simulink model "MPC_Demo_wuguzhang"  (R2024a)
settings: Solver=ode1  StartTime=0.001  StopTime=16  FixedStep=0.001  RelTol=1e-3  EnableMultiTasking=on
model workspace (MAT data in the model file):
  cc = 10
libraries: simulink x3, SignalEditorBlockLib x3, Solver_SF x1, slpidlib x1
(part 5 of 5)

== matlab function MPC_Demo_wuguzhang/Controller/MATLAB Function ==
  data: Vx input; beta output; Vy input; omega_1 input; omega_2 input; omega_3 input; omega_4 input; lamda1 output; lamda2 output; lamda3 output; lamda4 output
function [beta,lamda1,lamda2,lamda3,lamda4]= fct(Vx,Vy,omega_1,omega_2,omega_3,omega_4)
beta=-Vy/Vx;
Rw=0.393;
lamda1= (Rw *omega_1-Vx) / max(Vx, Rw *omega_1);
lamda2= (Rw *omega_2-Vx) / max(Vx, Rw *omega_2);
lamda3= (Rw *omega_3-Vx) / max(Vx, Rw *omega_3);
lamda4= (Rw *omega_4-Vx) / max(Vx, Rw *omega_4);

== matlab function MPC_Demo_wuguzhang/MATLAB Function5 ==
  data: Tor_L1 output; Tor_R1 output; Tor_L2 output; Tor_R2 output; Drive_torque input
function [Tor_L1,Tor_R1,Tor_L2,Tor_R2] = fcn(Drive_torque)

%L2左轮到右轮宽度
%deltaMxL1,deltaMxL2,deltaMxR1,deltaMxR2:分别是前左，后左，前右，后右的附加横摆力矩增量。和驱动力使用的驱动力矩相加就是总的轮胎力
%Rwheel,轮胎滚动半径


Tor_L1 = 0.25*Drive_torque;
Tor_L2 = 0.25*Drive_torque;
Tor_R1 = 0.25*Drive_torque;
Tor_R2 = 0.25*Drive_torque;

== matlab function MPC_Demo_wuguzhang/参考模型模块3/MATLAB Function ==
  data: Vx input; a output; b output; Tao_gama output; Tao_beta output; G_gama output; G_beta output; m input; I_z input; L input; L_f input; L_r input; C_f input; C_r input
function [a,b,Tao_gama,Tao_beta,G_gama,G_beta]  = para_cal_fcn(Vx, m, I_z, L, L_f, L_r, C_f, C_r)
%#codegen
K=(m*(C_f*L_f-C_r*L_r))/(2*L^2*C_f*C_r);
omga_n=(2*L/Vx)*sqrt((C_f*C_r*(1-K*Vx^2))/(m*I_z));
kesi=(m*(C_f*L_f^2+C_r*L_r^2)+(C_f+C_r)*I_z)/(2*L*sqrt(m*I_z*C_f*C_r*(1-K*Vx^2)));
tao_gama=(m*Vx*L_f)/(2*C_r*L);
g_gama=Vx/(L*(1-K*Vx^2));
tao_beta=(I_z*Vx)/(2*C_r*L_r*L-m*Vx^2*L_f);
g_beta=(2*L*L_r*C_r-m*Vx^2*L_f)/(2*L^2*C_r*(1-K*Vx^2));

a=1/(omga_n^2);
b=(2*kesi)/omga_n;
Tao_gama=tao_gama;
Tao_beta=tao_beta;
G_gama=g_gama;
G_beta=g_beta;

== matlab function MPC_Demo_wuguzhang/参考模型模块3/横摆角速度参考模型/MATLAB Function ==
  data: Vx input; wrd1 output; Steering1 input; Steering2 input; l input
function wrd1= fcn(Vx,Steering1,Steering2,l)
wrd1=Vx*(Steering1+Steering2)/2/(l+k_us_d*Vx*Vx);
end

== matlab function MPC_Demo_wuguzhang/参考模型模块3/横摆角速度参考模型/限幅模块/MATLAB Function ==
  data: mu input; wrd_max output; vx input; wrd1 input; wrd output
function [wrd_max,wrd]= fcn(mu,vx,wrd1)
%#eml
wrd_max=mu*9.8/(vx);


if abs(wrd1)<=abs(wrd_max)
    wrd=wrd1;
elseif wrd1>0
    wrd=abs(wrd_max);
else
    wrd=-abs(wrd_max);
end


end

== matlab function MPC_Demo_wuguzhang/参考模型模块3/质心侧偏角二阶参考模型/限幅模块 ==
  data: mu input; Vx input; beta_ref_sec output; beta_ref input; L_f input; L_r input; m input; C_f input; C_r input
function beta_ref_sec = fcn(mu,Vx,beta_ref, L_f, L_r, m, C_f, C_r)
%#codegen
% a=2*(L_f+L_r)*L_r*C_r*C_f;
% b=m*C_f*L_f*Vx^2;
% c=2*(L_f+L_r)^2*C_f*C_r-m*Vx^2*(L_f*C_f-L_r*C_r);
% beta_mid=((a-b)/c)*delta;
thre=mu*9.8*(L_r/Vx^2+m*L_f/(C_r*(L_f+L_r)));
if abs(beta_ref)>abs(thre)
    if beta_ref>=0
        beta_ref=abs(thre);
    else
        beta_ref=-abs(thre);
    end
    else
        beta_ref=beta_ref;
end

beta_ref_sec = beta_ref;

== matlab function MPC_Demo_wuguzhang/参考值生成模块/Target_Yawrate/MATLAB Function ==
  data: CarSimOut_Speed_ms input; Target_Yawrate_rads output; Lf input; Lr input; Ktar input; wheelAngle_rads input
function Target_Yawrate_rads  = VehicleModel_FrequPara(CarSimOut_Speed_ms,Lf,Lr,Ktar,wheelAngle_rads)


Target_Yawrate_rads=CarSimOut_Speed_ms/(CarSimOut_Speed_ms^2*Ktar*(Lf+Lr)+(Lf+Lr))*wheelAngle_rads;

== matlab function MPC_Demo_wuguzhang/参考模型模块/横摆角速度参考模型/MATLAB Function ==
  data: Vx input; wrd1 output; Steering1 input; Steering2 input; l input
function wrd1= fcn(Vx,Steering1,Steering2,l)
wrd1=Vx*(Steering1+Steering2)/2/(l+k_us_d*Vx*Vx);
end

== matlab function MPC_Demo_wuguzhang/参考值生成模块/Subsystem/MATLAB Function ==
  data: mu input; wrd_max output; vx input; wrd1 input; wrd output
function [wrd_max,wrd]= fcn(mu,vx,wrd1)
%#eml
wrd_max=mu.*9.8./(vx);


if abs(wrd1)<=abs(wrd_max)
    wrd=wrd1;
elseif wrd1>0
    wrd=abs(wrd_max);
else
    wrd=-abs(wrd_max);
end


end

== matlab function MPC_Demo_wuguzhang/MATLAB Function1 ==
  data: Vx input; beta output; Vy input; omega_1 input; omega_2 input; omega_3 input; omega_4 input; lamda1 output; lamda2 output; lamda3 output; lamda4 output
function [beta, lamda1, lamda2, lamda3, lamda4] = fct(Vx, Vy, omega_1, omega_2, omega_3, omega_4)
% 正常驾驶加速-减速过程曲线拟合（含可控滑移）
% 时间：0~16秒，起始速度12m/s，终止速度10m/s
% 设计原则：急加速+急减速，峰值滑移率≈20%（μ=0.7路面）

%% 1. 参数设置
dt = 0.1;                % 时间步长
t = 0:dt:16;             % 时间向量（0-16秒）
mu = 0.7;                % 路面摩擦系数（湿滑路面）
g = 9.81;                % 重力加速度
max_slip = 0.20;         % 允许最大滑移率（20%）
a_max = mu * g * max_slip; % 理论最大加速度 ≈1.37m/s²

%% 2. 生成速度曲线（三次样条插值控制点）
% 控制点：时间 [0, 4, 8, 12, 16] 秒
%         速度 [12, 20, 25, 18, 10] m/s
ctrl_time = [0, 4, 8, 12, 16];
ctrl_vel = [12, 20, 25, 18, 10];

% 三次样条插值
vel = spline(ctrl_time, ctrl_vel, t);

%% 3. 计算加速度
acc = diff(vel)/dt;         % 加速度（差分近似）
t_acc = t(1:end-1) + dt/2;  % 加速度对应的时间点

%% 4. 计算理论滑移率
slip_ratio = abs(acc) / (mu * g);  % 滑移率 = |加速度| / (μ·g)

%% 5. 可视化结果
figure('Position', [100, 100, 800, 600])

% 速度曲线
subplot(3,1,1);
plot(t, vel, 'b-', 'LineWidth', 2);
hold on;
plot(ctrl_time, ctrl_vel, 'ro', 'MarkerSize', 8, 'LineWidth', 2);
title('速度-时间曲线');
xlabel('时间 (s)');
ylabel('速度 (m/s)');
legend('实际速度', '控制点', 'Location', 'northwest');
grid on;
xlim([0,16]);
ylim([0,30]);

% 加速度曲线
subplot(3,1,2);
plot(t_acc, acc, 'r-', 'LineWidth', 1.5);
hold on;
yline(a_max, '--k', 'Max Accel', 'LineWidth', 1.2);
yline(-a_max, '--k', 'Max Decel', 'LineWidth', 1.2);
title('加速度-时间曲线');
xlabel('时间 (s)');
ylabel('加速度 (m/s²)');
grid on;
xlim([0,16]);
ylim([-3, 3]);

% 滑移率曲线
subplot(3,1,3);
plot(t_acc, slip_ratio*100, 'm-', 'LineWidth', 1.5);
hold on;
yline(max_slip*100, '--r', '安全阈值 (20%)', 'LineWidth', 1.5);
title('轮胎滑移率');
xlabel('时间 (s)');
ylabel('滑移率 (%)');
grid on;
xlim([0,16]);
ylim([0, 30]);

%% 6. 输出关键指标
fprintf('驾驶过程分析 (μ=%.1f路面):\n', mu);
fprintf('最大加速度: %.2f m/s² (%.1f%% 滑移率)\n',...
    max(acc), max(slip_ratio)*100);
fprintf('最大减速度: %.2f m/s² (%.1f%% 滑移率)\n',...
    abs(min(acc)), max(slip_ratio)*100);
fprintf('加速阶段: 0-8秒, %.1f → %.1f m/s\n', vel(1), vel(find(t>=8,1)));
fprintf('减速阶段: 8-16秒, %.1f → %.1f m/s\n', vel(find(t>=8,1)), vel(end));

== matlab function MPC_Demo_wuguzhang/参考值生成模块/质心侧偏角参考值生成 ==
  data: mu input; Vx input; beta_ref output; delta input; L_f input; L_r input; m input; C_f input; C_r input
function beta_ref = fcn(mu,Vx,delta, L_f, L_r, m, C_f, C_r)
%#codegen
a=2*(L_f+L_r)*L_r*C_r*C_f;
b=m*C_f*L_f*Vx^2;
c=2*(L_f+L_r)^2*C_f*C_r-m*Vx^2*(L_f*C_f-L_r*C_r);
beta_mid=((a-b)/c)*delta;
thre=mu*9.8*(L_r/Vx^2+m*L_f/(C_r*(L_f+L_r)));
if abs(beta_mid)>abs(thre)
    if beta_mid>=0
        beta_mid=abs(thre);
    else
        beta_mid=-abs(thre);
    end
    else
        beta_mid=beta_mid;
end

beta_ref = beta_mid;

== matlab function MPC_Demo_wuguzhang/参考模型模块/MATLAB Function ==
  data: Vx input; a output; b output; Tao_gama output; Tao_beta output; G_gama output; G_beta output; m input; I_z input; L input; L_f input; L_r input; C_f input; C_r input
function [a,b,Tao_gama,Tao_beta,G_gama,G_beta]  = para_cal_fcn(Vx, m, I_z, L, L_f, L_r, C_f, C_r)
%#codegen
K=(m*(C_f*L_f-C_r*L_r))/(2*L^2*C_f*C_r);
omga_n=(2*L/Vx)*sqrt((C_f*C_r*(1-K*Vx^2))/(m*I_z));
kesi=(m*(C_f*L_f^2+C_r*L_r^2)+(C_f+C_r)*I_z)/(2*L*sqrt(m*I_z*C_f*C_r*(1-K*Vx^2)));
tao_gama=(m*Vx*L_f)/(2*C_r*L);
g_gama=Vx/(L*(1-K*Vx^2));
tao_beta=(I_z*Vx)/(2*C_r*L_r*L-m*Vx^2*L_f);
g_beta=(2*L*L_r*C_r-m*Vx^2*L_f)/(2*L^2*C_r*(1-K*Vx^2));

a=1/(omga_n^2);
b=(2*kesi)/omga_n;
Tao_gama=tao_gama;
Tao_beta=tao_beta;
G_gama=g_gama;
G_beta=g_beta;
